simulink library "WECSim_Lib"  (R2014b)
settings: Solver=ode45  StartTime=0.0  StopTime=10.0  RelTol=1e-3
undefined symbols (not defined in the file): body, constraint, pto, simu, waves, X, Y, Z
libraries: nesl_utility x178, sm_lib x59, vrlib x12
(part 2 of 6)

== system WECSim_Lib/Constraints/Heave ==
  note: Constraints the motion to the desired DOF.
      | Moves the connection points (B and F) from the free surface to the PTO location.
      | Outputs forces and motions.
  note: constraint.loc
      | constraint.c
      | constraint.k
      | constraint.name used in mask
  Add : Sum
  "Assignment (3rd index) " : Assignment  Indices=3
  Assignment (3rd index)1 : Assignment  Indices=3
  Assignment (3rd index)2 : Assignment  Indices=3
  Constant{,1..3} (4 alike) : Constant  Value=[0 0 0 0 0 0]
  Initial Displacement and Angle : Constant  Value=constraint.mooring.initLinDispAngle
  Mooring : Subsystem  Variant=on
  Mux : Mux  Inputs=2
  Mux1 : Mux  Inputs=6
  Mux2 : Mux  Inputs=2
  PS-Simulink Converter{,1..6} (7 alike) : nesl_utility/PS-Simulink Converter  PhysicalDomain=network_engine_domain  SubClassName=ps_output  LeftPortType=input  RightPortType=output  PseudoPeriodic=off  Frequencies=[]  Unit=1  AffineConversion=off
  Prismatic Joint (Translational Constraint) : sm_lib/Joints/Prismatic Joint  SenseConstraintForce=on  SenseConstraintForceX=off  SenseConstraintForceY=off  SenseConstraintForceZ=off  SenseConstraintTorque=on  SenseConstraintTorqueX=off  SenseConstraintTorqueY=off  SenseConstraintTorqueZ=off  SenseTotalForce=on  SenseTotalForceX=off  SenseTotalForceY=off  SenseTotalForceZ=off  SenseTotalTorque=on  SenseTotalTorqueX=off  SenseTotalTorqueY=off  SenseTotalTorqueZ=off  CompositeWrenchDir=BaseOnFollower  CompositeWrenchFrame=BaseFrame  EquilibriumPosition=0  EquilibriumPositionUnits=m  SpringStiffness=0  SpringStiffnessUnits=N/m  DampingCoefficient=0  DampingCoefficientUnits=N/(m/s)  TorqueActuationMode=InputTorque  MotionActuationMode=ComputedMotion  SensePosition=on  SenseVelocity=on  SenseAcceleration=on  SenseTorqueForce=off  PositionTargetValue=0  PositionTargetValueUnits=m  PositionTargetSpecify=off  PositionTargetPriority=High  VelocityTargetValue=0  VelocityTargetValueUnits=m/s  VelocityTargetSpecify=off  VelocityTargetPriority=High  BlockFunction=simmechanics.library.joints.prismatic_joint
  Rigid Transform : sm_lib/Frames and Transforms/Rigid Transform  TranslationMethod=Cartesian  TranslationLengthUnit=m  TranslationStandardAxis=+Z  TranslationStandardOffset=0  TranslationCartesianOffset=constraint.loc  TranslationROffset=0  TranslationROffsetUnits=m  TranslationZOffset=0  TranslationZOffsetUnits=m  TranslationThetaOffset=0  TranslationThetaOffsetUnits=deg  RotationMethod=None  RotationAngleUnits=deg  RotationStandardAxis=+X  RotationAngle=90  RotationArbitraryAxis=[0 0 1]  FollAlignAxisA=+X  BaseAlignAxisA=+Y  FollAlignAxisB=+Y  BaseAlignAxisB=+Z  RotationMatrix=[1 0 0; 0 1 0; 0 0 1]  BlockFunction=simmechanics.library.frames_transforms.rigid_transform
  Rigid Transform1 : sm_lib/Frames and Transforms/Rigid Transform  TranslationMethod=Cartesian  TranslationLengthUnit=m  TranslationStandardAxis=+Z  TranslationStandardOffset=0  TranslationCartesianOffset=constraint.loc  TranslationROffset=0  TranslationROffsetUnits=m  TranslationZOffset=0  TranslationZOffsetUnits=m  TranslationThetaOffset=0  TranslationThetaOffsetUnits=deg  RotationMethod=None  RotationAngleUnits=deg  RotationStandardAxis=+X  RotationAngle=90  RotationArbitraryAxis=[0 0 1]  FollAlignAxisA=+X  BaseAlignAxisA=+Y  FollAlignAxisB=+Y  BaseAlignAxisB=+Z  RotationMatrix=[1 0 0; 0 1 0; 0 0 1]  BlockFunction=simmechanics.library.frames_transforms.rigid_transform
  Selector2 : Selector  InputPortWidth=6  Indices=3
  Simulink-PS Converter2 : nesl_utility/Simulink-PS Converter  PhysicalDomain=network_engine_domain  SubClassName=ps_input  LeftPortType=input  RightPortType=output  PseudoPeriodic=off  Frequencies=[]  NoiseDistribution=none  NoiseParameters=[]  Unit=1  AffineConversion=off  InputFiltering=off  SimscapeFilterOrder=1  InputFilterTimeConstant=0.001  UdotUserProvided=1
  output : ToWorkspace  VariableName=constraint1_out  SaveFormat=Structure With Time  SampleTime=-1
      settings: Decimation=round(simu.dtOut/simu.dt,0)
  F : PMIOPort  Port=1  Side=Right
  B : PMIOPort  Port=2  Side=Left
  wires:
  Mux1/1 -> output/1
  Assignment (3rd index)2/1 -> Mux1/3  "acceleration"
  Constant/1 -> "Assignment (3rd index) "/1
  PS-Simulink Converter2/1 -> "Assignment (3rd index) "/2
  Constant1/1 -> Assignment (3rd index)1/1
  PS-Simulink Converter3/1 -> Assignment (3rd index)1/2
  Constant2/1 -> Assignment (3rd index)2/1
  PS-Simulink Converter4/1 -> Assignment (3rd index)2/2
  Mux/1 -> Mux1/5  "Constraint Forces"
  PS-Simulink Converter1/1 -> Mux/2
  PS-Simulink Converter/1 -> Mux/1
  Mux2/1 -> Mux1/4  "Total Forces"
  PS-Simulink Converter6/1 -> Mux2/2
  PS-Simulink Converter5/1 -> Mux2/1
  Constant3/1 -> Mux1/6  "Mooring Forces"
  Assignment (3rd index)1/1 -> Mooring/3(Velocity), Mux1/2  "velocity"
  "Assignment (3rd index) "/1 -> Add/1, Mux1/1  "position"
  Mooring/1(F_Mooring) -> Selector2/1
  Selector2/1 -> Simulink-PS Converter2/1
  [Clock] -> Mooring/2(Clock)
  Initial Displacement and Angle/1 -> Add/2
  Add/1 -> Mooring/1(Displacement)
  connections:
  PS-Simulink Converter1/LConn1 -- Prismatic Joint (Translational Constraint)/RConn6
  Prismatic Joint (Translational Constraint)/RConn5 -- PS-Simulink Converter/LConn1
  PS-Simulink Converter4/LConn1 -- Prismatic Joint (Translational Constraint)/RConn4
  PS-Simulink Converter3/LConn1 -- Prismatic Joint (Translational Constraint)/RConn3
  PS-Simulink Converter2/LConn1 -- Prismatic Joint (Translational Constraint)/RConn2
  Rigid Transform/RConn1 -- Prismatic Joint (Translational Constraint)/LConn1
  B/RConn1 -- Rigid Transform/LConn1
  Rigid Transform1/LConn1 -- F/RConn1
  Rigid Transform1/RConn1 -- Prismatic Joint (Translational Constraint)/RConn1
  Prismatic Joint (Translational Constraint)/RConn7 -- PS-Simulink Converter5/LConn1
  Prismatic Joint (Translational Constraint)/RConn8 -- PS-Simulink Converter6/LConn1
  Simulink-PS Converter2/RConn1 -- Prismatic Joint (Translational Constraint)/LConn2

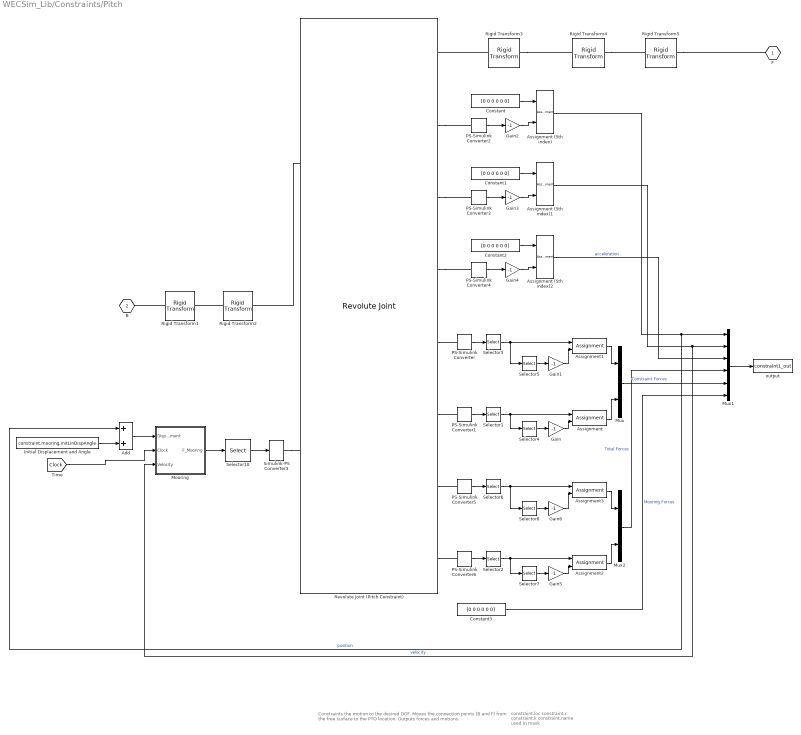
== system WECSim_Lib/Constraints/Pitch ==
  note: constraint.loc
      | constraint.c
      | constraint.k
      | constraint.name used in mask
  note: Constraints the motion to the desired DOF.
      | Moves the connection points (B and F) from the free surface to the PTO location.
      | Outputs forces and motions.
  Add : Sum
  Assignment{,1..3} (4 alike) : Assignment  DiagnosticForDimensions=Warning  Indices=2
  "Assignment (5th index) " : Assignment  Indices=5
  Assignment (5th index)1 : Assignment  Indices=5
  Assignment (5th index)2 : Assignment  Indices=5
  Constant{,1..3} (4 alike) : Constant  Value=[0 0 0 0 0 0]
  Gain{,1..6} (7 alike) : Gain  Gain=-1
  Initial Displacement and Angle : Constant  Value=constraint.mooring.initLinDispAngle
  Mooring : Subsystem  Variant=on
  Mux : Mux  Inputs=2
  Mux1 : Mux  Inputs=6
  Mux2 : Mux  Inputs=2
  PS-Simulink Converter{,1..6} (7 alike) : nesl_utility/PS-Simulink Converter  PhysicalDomain=network_engine_domain  SubClassName=ps_output  LeftPortType=input  RightPortType=output  PseudoPeriodic=off  Frequencies=[]  Unit=1  AffineConversion=off
  Revolute Joint (Pitch Constraint) : sm_lib/Joints/Revolute Joint  SenseConstraintForce=on  SenseConstraintForceX=off  SenseConstraintForceY=off  SenseConstraintForceZ=off  SenseConstraintTorque=on  SenseConstraintTorqueX=off  SenseConstraintTorqueY=off  SenseConstraintTorqueZ=off  SenseTotalForce=on  SenseTotalForceX=off  SenseTotalForceY=off  SenseTotalForceZ=off  SenseTotalTorque=on  SenseTotalTorqueX=off  SenseTotalTorqueY=off  SenseTotalTorqueZ=off  CompositeWrenchDir=BaseOnFollower  CompositeWrenchFrame=BaseFrame  EquilibriumPosition=0  EquilibriumPositionUnits=deg  SpringStiffness=0  SpringStiffnessUnits=N*m/deg  DampingCoefficient=0  DampingCoefficientUnits=N*m/(rad/s)  TorqueActuationMode=InputTorque  MotionActuationMode=ComputedMotion  SensePosition=on  SenseVelocity=on  SenseAcceleration=on  SenseTorqueForce=off  PositionTargetValue=0  PositionTargetValueUnits=deg  PositionTargetSpecify=off  PositionTargetPriority=High  VelocityTargetValue=0  VelocityTargetValueUnits=deg/s  VelocityTargetSpecify=off  VelocityTargetPriority=High  BlockFunction=simmechanics.library.joints.revolute_joint
  Rigid Transform1 : sm_lib/Frames and Transforms/Rigid Transform  TranslationMethod=Cartesian  TranslationLengthUnit=m  TranslationStandardAxis=+Z  TranslationStandardOffset=0  TranslationCartesianOffset=constraint.loc  TranslationROffset=0  TranslationROffsetUnits=m  TranslationZOffset=0  TranslationZOffsetUnits=m  TranslationThetaOffset=0  TranslationThetaOffsetUnits=deg  RotationMethod=None  RotationAngleUnits=deg  RotationStandardAxis=+X  RotationAngle=90  RotationArbitraryAxis=[0 0 1]  FollAlignAxisA=+X  BaseAlignAxisA=+Y  FollAlignAxisB=+Y  BaseAlignAxisB=+Z  RotationMatrix=[1 0 0; 0 1 0; 0 0 1]  BlockFunction=simmechanics.library.frames_transforms.rigid_transform
  Rigid Transform2 : sm_lib/Frames and Transforms/Rigid Transform  TranslationMethod=None  TranslationLengthUnit=m  TranslationStandardAxis=+Z  TranslationStandardOffset=0  TranslationCartesianOffset=[0 0 0]  TranslationROffset=0  TranslationROffsetUnits=m  TranslationZOffset=0  TranslationZOffsetUnits=m  TranslationThetaOffset=0  TranslationThetaOffsetUnits=deg  RotationMethod=StandardAxis  RotationAngleUnits=deg  RotationStandardAxis=+X  RotationAngle=90  RotationArbitraryAxis=[0 0 1]  FollAlignAxisA=+X  BaseAlignAxisA=+Y  FollAlignAxisB=+Y  BaseAlignAxisB=+Z  RotationMatrix=[1 0 0; 0 1 0; 0 0 1]  BlockFunction=simmechanics.library.frames_transforms.rigid_transform
  Rigid Transform3 : sm_lib/Frames and Transforms/Rigid Transform  TranslationMethod=None  TranslationLengthUnit=m  TranslationStandardAxis=+Z  TranslationStandardOffset=0  TranslationCartesianOffset=constraint.loc  TranslationROffset=0  TranslationROffsetUnits=m  TranslationZOffset=0  TranslationZOffsetUnits=m  TranslationThetaOffset=0  TranslationThetaOffsetUnits=deg  RotationMethod=StandardAxis  RotationAngleUnits=rad  RotationStandardAxis=-Z  RotationAngle=constraint.initDisp  RotationArbitraryAxis=[0 0 1]  FollAlignAxisA=+X  BaseAlignAxisA=+Y  FollAlignAxisB=+Y  BaseAlignAxisB=+Z  RotationMatrix=[1 0 0; 0 1 0; 0 0 1]  BlockFunction=simmechanics.library.frames_transforms.rigid_transform
  Rigid Transform4 : sm_lib/Frames and Transforms/Rigid Transform  TranslationMethod=None  TranslationLengthUnit=m  TranslationStandardAxis=+Z  TranslationStandardOffset=0  TranslationCartesianOffset=constraint.loc  TranslationROffset=0  TranslationROffsetUnits=m  TranslationZOffset=0  TranslationZOffsetUnits=m  TranslationThetaOffset=0  TranslationThetaOffsetUnits=deg  RotationMethod=StandardAxis  RotationAngleUnits=deg  RotationStandardAxis=+X  RotationAngle=-90  RotationArbitraryAxis=[0 0 1]  FollAlignAxisA=+X  BaseAlignAxisA=+Y  FollAlignAxisB=+Y  BaseAlignAxisB=+Z  RotationMatrix=[1 0 0; 0 1 0; 0 0 1]  BlockFunction=simmechanics.library.frames_transforms.rigid_transform
  Rigid Transform5 : sm_lib/Frames and Transforms/Rigid Transform  TranslationMethod=Cartesian  TranslationLengthUnit=m  TranslationStandardAxis=+Z  TranslationStandardOffset=0  TranslationCartesianOffset=[-constraint.loc(1)*cos(-constraint.initDisp)-constraint.loc(3)*sin(-constraint.initDisp), 0, constraint.loc(1)*sin(-constraint.initDisp)-constraint.loc(3)*cos(-constraint.initDisp)]  TranslationROffset=0  TranslationROffsetUnits=m  TranslationZOffset=0  TranslationZOffsetUnits=m  TranslationThetaOffset=0  TranslationThetaOffsetUnits=deg  RotationMethod=None  RotationAngleUnits=deg  RotationStandardAxis=+X  RotationAngle=-90  RotationArbitraryAxis=[0 0 1]  FollAlignAxisA=+X  BaseAlignAxisA=+Y  FollAlignAxisB=+Y  BaseAlignAxisB=+Z  RotationMatrix=[1 0 0; 0 1 0; 0 0 1]  BlockFunction=simmechanics.library.frames_transforms.rigid_transform
  Selector{1..3,6} (4 alike) : Selector  InputPortWidth=3  Indices=[1 3 2]
  Selector10 : Selector  InputPortWidth=6  Indices=5
  Selector{4..5,7..8} (4 alike) : Selector  InputPortWidth=3  Indices=[2]
  Simulink-PS Converter3 : nesl_utility/Simulink-PS Converter  PhysicalDomain=network_engine_domain  SubClassName=ps_input  LeftPortType=input  RightPortType=output  PseudoPeriodic=off  Frequencies=[]  NoiseDistribution=none  NoiseParameters=[]  Unit=1  AffineConversion=off  InputFiltering=off  SimscapeFilterOrder=1  InputFilterTimeConstant=0.001  UdotUserProvided=1
  output : ToWorkspace  VariableName=constraint1_out  SaveFormat=Structure With Time  SampleTime=-1
      settings: Decimation=round(simu.dtOut/simu.dt,0)
  F : PMIOPort  Port=1  Side=Right
  B : PMIOPort  Port=2  Side=Left
  wires:
  Constant3/1 -> Mux1/6  "Mooring Forces"
  PS-Simulink Converter5/1 -> Selector6/1
  PS-Simulink Converter6/1 -> Selector2/1
  Selector2/1 -> Assignment2/1, Selector7/1
  Selector7/1 -> Gain5/1
  Gain5/1 -> Assignment2/2
  Selector6/1 -> Assignment3/1, Selector8/1
  Selector8/1 -> Gain6/1
  Gain6/1 -> Assignment3/2
  Assignment3/1 -> Mux2/1
  Assignment2/1 -> Mux2/2
  Mux2/1 -> Mux1/4  "Total Forces"
  PS-Simulink Converter/1 -> Selector3/1
  PS-Simulink Converter1/1 -> Selector1/1
  Selector1/1 -> Selector4/1, Assignment/1
  Selector4/1 -> Gain/1
  Gain/1 -> Assignment/2
  Selector3/1 -> Selector5/1, Assignment1/1
  Selector5/1 -> Gain1/1
  Gain1/1 -> Assignment1/2
  Assignment1/1 -> Mux/1
  Assignment (5th index)2/1 -> Mux1/3  "acceleration"
  Gain4/1 -> Assignment (5th index)2/2
  Constant2/1 -> Assignment (5th index)2/1
  PS-Simulink Converter4/1 -> Gain4/1
  PS-Simulink Converter3/1 -> Gain3/1
  Gain3/1 -> Assignment (5th index)1/2
  Constant1/1 -> Assignment (5th index)1/1
  Gain2/1 -> "Assignment (5th index) "/2
  PS-Simulink Converter2/1 -> Gain2/1
  Constant/1 -> "Assignment (5th index) "/1
  Assignment/1 -> Mux/2
  Mux1/1 -> output/1
  Mux/1 -> Mux1/5  "Constraint Forces"
  Assignment (5th index)1/1 -> Mooring/3(Velocity), Mux1/2  "velocity"
  "Assignment (5th index) "/1 -> Add/1, Mux1/1  "position"
  Mooring/1(F_Mooring) -> Selector10/1
  Selector10/1 -> Simulink-PS Converter3/1
  [Clock] -> Mooring/2(Clock)
  Initial Displacement and Angle/1 -> Add/2
  Add/1 -> Mooring/1(Displacement)
  connections:
  Rigid Transform5/RConn1 -- F/RConn1
  Rigid Transform4/RConn1 -- Rigid Transform5/LConn1
  Rigid Transform3/RConn1 -- Rigid Transform4/LConn1
  PS-Simulink Converter6/LConn1 -- Revolute Joint (Pitch Constraint)/RConn8
  PS-Simulink Converter5/LConn1 -- Revolute Joint (Pitch Constraint)/RConn7
  Rigid Transform2/LConn1 -- Rigid Transform1/RConn1
  Revolute Joint (Pitch Constraint)/LConn1 -- Rigid Transform2/RConn1
  PS-Simulink Converter/LConn1 -- Revolute Joint (Pitch Constraint)/RConn5
  PS-Simulink Converter1/LConn1 -- Revolute Joint (Pitch Constraint)/RConn6
  Revolute Joint (Pitch Constraint)/RConn2 -- PS-Simulink Converter2/LConn1
  Revolute Joint (Pitch Constraint)/RConn3 -- PS-Simulink Converter3/LConn1
  Revolute Joint (Pitch Constraint)/RConn4 -- PS-Simulink Converter4/LConn1
  Rigid Transform3/LConn1 -- Revolute Joint (Pitch Constraint)/RConn1
  Rigid Transform1/LConn1 -- B/RConn1
  Simulink-PS Converter3/RConn1 -- Revolute Joint (Pitch Constraint)/LConn2

== system WECSim_Lib/Constraints/Surge ==
  note: Constraints the motion to the desired DOF.
      | Moves the connection points (B and F) from the free surface to the PTO location.
      | Outputs forces and motions.
  note: constraint.loc
      | constraint.c
      | constraint.k
      | constraint.name used in mask
  Add : Sum
  Assignment{,1..3} (4 alike) : Assignment  DiagnosticForDimensions=Warning  Indices=3
  "Assignment (1st index) " : Assignment
  Assignment (1st index)1 : Assignment
  Assignment (1st index)2 : Assignment
  Constant{,1..3} (4 alike) : Constant  Value=[0 0 0 0 0 0]
  Gain{,1..3} (4 alike) : Gain  Gain=-1
  Initial Displacement and Angle : Constant  Value=constraint.mooring.initLinDispAngle
  Mooring : Subsystem  Variant=on
  Mux : Mux  Inputs=2
  Mux1 : Mux  Inputs=6
  Mux2 : Mux  Inputs=2
  PS-Simulink Converter{1..7} (7 alike) : nesl_utility/PS-Simulink Converter  PhysicalDomain=network_engine_domain  SubClassName=ps_output  LeftPortType=input  RightPortType=output  PseudoPeriodic=off  Frequencies=[]  Unit=1  AffineConversion=off
  Prismatic Joint (Translational Constraint) : sm_lib/Joints/Prismatic Joint  SenseConstraintForce=on  SenseConstraintForceX=off  SenseConstraintForceY=off  SenseConstraintForceZ=off  SenseConstraintTorque=on  SenseConstraintTorqueX=off  SenseConstraintTorqueY=off  SenseConstraintTorqueZ=off  SenseTotalForce=on  SenseTotalForceX=off  SenseTotalForceY=off  SenseTotalForceZ=off  SenseTotalTorque=on  SenseTotalTorqueX=off  SenseTotalTorqueY=off  SenseTotalTorqueZ=off  CompositeWrenchDir=BaseOnFollower  CompositeWrenchFrame=BaseFrame  EquilibriumPosition=0  EquilibriumPositionUnits=m  SpringStiffness=0  SpringStiffnessUnits=N/m  DampingCoefficient=0  DampingCoefficientUnits=N/(m/s)  TorqueActuationMode=InputTorque  MotionActuationMode=ComputedMotion  SensePosition=on  SenseVelocity=on  SenseAcceleration=on  SenseTorqueForce=off  PositionTargetValue=0  PositionTargetValueUnits=m  PositionTargetSpecify=off  PositionTargetPriority=High  VelocityTargetValue=0  VelocityTargetValueUnits=m/s  VelocityTargetSpecify=off  VelocityTargetPriority=High  BlockFunction=simmechanics.library.joints.prismatic_joint
  Rigid Transform : sm_lib/Frames and Transforms/Rigid Transform  TranslationMethod=Cartesian  TranslationLengthUnit=m  TranslationStandardAxis=+Z  TranslationStandardOffset=0  TranslationCartesianOffset=constraint.loc  TranslationROffset=0  TranslationROffsetUnits=m  TranslationZOffset=0  TranslationZOffsetUnits=m  TranslationThetaOffset=0  TranslationThetaOffsetUnits=deg  RotationMethod=StandardAxis  RotationAngleUnits=deg  RotationStandardAxis=+Y  RotationAngle=90  RotationArbitraryAxis=[0 0 1]  FollAlignAxisA=+X  BaseAlignAxisA=+Y  FollAlignAxisB=+Y  BaseAlignAxisB=+Z  RotationMatrix=[1 0 0; 0 1 0; 0 0 1]  BlockFunction=simmechanics.library.frames_transforms.rigid_transform
  Rigid Transform1 : sm_lib/Frames and Transforms/Rigid Transform  TranslationMethod=Cartesian  TranslationLengthUnit=m  TranslationStandardAxis=+Z  TranslationStandardOffset=0  TranslationCartesianOffset=constraint.loc  TranslationROffset=0  TranslationROffsetUnits=m  TranslationZOffset=0  TranslationZOffsetUnits=m  TranslationThetaOffset=0  TranslationThetaOffsetUnits=deg  RotationMethod=StandardAxis  RotationAngleUnits=deg  RotationStandardAxis=+Y  RotationAngle=90  RotationArbitraryAxis=[0 0 1]  FollAlignAxisA=+X  BaseAlignAxisA=+Y  FollAlignAxisB=+Y  BaseAlignAxisB=+Z  RotationMatrix=[1 0 0; 0 1 0; 0 0 1]  BlockFunction=simmechanics.library.frames_transforms.rigid_transform
  Selector : Selector  InputPortWidth=6
  Selector{1..2,5..6} (4 alike) : Selector  InputPortWidth=3  Indices=[3 2 1]
  Selector{3..4,7..8} (4 alike) : Selector  InputPortWidth=3  Indices=[3]
  Simulink-PS Converter1 : nesl_utility/Simulink-PS Converter  PhysicalDomain=network_engine_domain  SubClassName=ps_input  LeftPortType=input  RightPortType=output  PseudoPeriodic=off  Frequencies=[]  NoiseDistribution=none  NoiseParameters=[]  Unit=1  AffineConversion=off  InputFiltering=off  SimscapeFilterOrder=1  InputFilterTimeConstant=0.001  UdotUserProvided=1
  output : ToWorkspace  VariableName=constraint1_out  SaveFormat=Structure With Time  SampleTime=-1
      settings: Decimation=round(simu.dtOut/simu.dt,0)
  F : PMIOPort  Port=1  Side=Right
  B : PMIOPort  Port=2  Side=Left
  wires:
  Mux1/1 -> output/1
  Assignment (1st index)2/1 -> Mux1/3  "acceleration"
  Constant/1 -> "Assignment (1st index) "/1
  PS-Simulink Converter2/1 -> "Assignment (1st index) "/2
  Constant1/1 -> Assignment (1st index)1/1
  PS-Simulink Converter3/1 -> Assignment (1st index)1/2
  Constant2/1 -> Assignment (1st index)2/1
  PS-Simulink Converter4/1 -> Assignment (1st index)2/2
  PS-Simulink Converter5/1 -> Selector2/1
  PS-Simulink Converter1/1 -> Selector1/1
  Assignment1/1 -> Mux/1
  Assignment/1 -> Mux/2
  Gain1/1 -> Assignment1/2
  Selector3/1 -> Gain1/1
  Selector2/1 -> Assignment1/1, Selector3/1
  Gain/1 -> Assignment/2
  Selector4/1 -> Gain/1
  Selector1/1 -> Assignment/1, Selector4/1
  Mux/1 -> Mux1/5  "Constraint Forces"
  Constant3/1 -> Mux1/6  "Mooring Forces"
  PS-Simulink Converter7/1 -> Selector6/1
  PS-Simulink Converter6/1 -> Selector5/1
  Assignment3/1 -> Mux2/1
  Assignment2/1 -> Mux2/2
  Gain3/1 -> Assignment3/2
  Selector7/1 -> Gain3/1
  Selector6/1 -> Assignment3/1, Selector7/1
  Gain2/1 -> Assignment2/2
  Selector8/1 -> Gain2/1
  Selector5/1 -> Assignment2/1, Selector8/1
  Mux2/1 -> Mux1/4  "Total Forces"
  Assignment (1st index)1/1 -> Mooring/3(Velocity), Mux1/2  "velocity"
  "Assignment (1st index) "/1 -> Add/1, Mux1/1  "position"
  Mooring/1(F_Mooring) -> Selector/1
  [Clock] -> Mooring/2(Clock)
  Initial Displacement and Angle/1 -> Add/2
  Add/1 -> Mooring/1(Displacement)
  Selector/1 -> Simulink-PS Converter1/1
  connections:
  F/RConn1 -- Rigid Transform1/LConn1
  PS-Simulink Converter1/LConn1 -- Prismatic Joint (Translational Constraint)/RConn6
  PS-Simulink Converter5/LConn1 -- Prismatic Joint (Translational Constraint)/RConn5
  PS-Simulink Converter2/LConn1 -- Prismatic Joint (Translational Constraint)/RConn2
  PS-Simulink Converter3/LConn1 -- Prismatic Joint (Translational Constraint)/RConn3
  PS-Simulink Converter4/LConn1 -- Prismatic Joint (Translational Constraint)/RConn4
  Rigid Transform/LConn1 -- B/RConn1
  Rigid Transform/RConn1 -- Prismatic Joint (Translational Constraint)/LConn1
  Rigid Transform1/RConn1 -- Prismatic Joint (Translational Constraint)/RConn1
  Prismatic Joint (Translational Constraint)/RConn7 -- PS-Simulink Converter7/LConn1
  Prismatic Joint (Translational Constraint)/RConn8 -- PS-Simulink Converter6/LConn1
  Simulink-PS Converter1/RConn1 -- Prismatic Joint (Translational Constraint)/LConn2

== system WECSim_Lib/Frames/Global Reference Frame ==
  note: simu.domainSize
      | waves.waterDepth
  note: Serves as the global reference frame for any WEC-Sim simulation.
      | Has a connection point at (0,0,0), defined at the free surface.
      | Sets up the free surface and ground visualization.
      | Sends the simulation time to a GoTo that can be accesed by other blocks.
  Clock : Clock
  Mean Free Surface : sm_lib/Body Elements/Solid  InertiaType=Custom  Mass=10^20  MassUnits=kg  CenterOfMass=[0 0 0]  CenterOfMassUnits=m  MomentsOfInertia=[10^20 10^20 10^20]  MomentsOfInertiaUnits=kg*m^2  ProductsOfInertia=[0 0 0]  ProductsOfInertiaUnits=kg*m^2  DensityBased=on  Density=1000  DensityUnits=kg/(m^3)  GraphicType=FromGeometry  MarkerShape=Sphere  MarkerSize=10  MarkerSizeUnits=m  GraphicVisPropType=SimpleVisualProperties  GraphicDiffuseColor=[0.0 0.6 0.8]  GraphicSpecularColor=[0.5 0.5 0.5 1.0]  GraphicAmbientColor=[0.15 0.15 0.15 1.0]  GraphicEmissiveColor=[0.0 0.0 0.0 1.0]  GraphicShininess=75  GraphicOpacity=0.3  GeometryShape=GeneralExtrusion  RectangleSize=[1 1]  RectangleSizeUnits=m  BrickDimensions=[1 1 1]  BrickDimensionUnits=m  CylinderRadius=1  CylinderRadiusUnits=m  CylinderLength=1  CylinderLengthUnits=m  SphereRadius=1  SphereRadiusUnits=m  EllipsoidRadii=[1 1 1]  EllipsoidRadiiUnits=m  ExtrusionCrossSection=[simu.domainSize simu.domainSize; -simu.domainSize simu.domainSize; -simu.domainSize -simu.domainSize; simu.domainSize -simu.domainSize]  ExtrusionCrossSectionUnits=m  ExtrusionLength=simu.domainSize/200  ExtrusionLengthUnits=m  PolygonNumSides=3  PolygonOuterRadius=1  PolygonOuterRadiusUnits=m  ExtGeomFileType=STL  ExtGeomFileUnits=m  RevolutionCrossSection=[1 1; 1 -1; 2 -1; 2 1]  RevolutionCrossSectionUnits=m  RevolutionExtent=Full  RevolutionAngle=180  RevolutionAngleUnits=deg  BlockFunction=simmechanics.library.body_elements.solid
  Mechanism Configuration : sm_lib/Utilities/Mechanism Configuration  UniformGravity=Constant  GravityVector=[0 0 0]  GravityUnits=m/s^2  LinearizationDelta=0.001  BlockFunction=simmechanics.library.utilities.mechanism_configuration
  Rigid Transform : sm_lib/Frames and Transforms/Rigid Transform  TranslationMethod=Cartesian  TranslationLengthUnit=m  TranslationStandardAxis=+Z  TranslationStandardOffset=0  TranslationCartesianOffset=[0 0 -waves.waterDepth]  TranslationROffset=0  TranslationROffsetUnits=m  TranslationZOffset=0  TranslationZOffsetUnits=m  TranslationThetaOffset=0  TranslationThetaOffsetUnits=deg  RotationMethod=None  RotationAngleUnits=deg  RotationStandardAxis=+Z  RotationAngle=0  RotationArbitraryAxis=[0 0 1]  FollAlignAxisA=+X  BaseAlignAxisA=+Y  FollAlignAxisB=+Y  BaseAlignAxisB=+Z  RotationMatrix=[1 0 0; 0 1 0; 0 0 1]  BlockFunction=simmechanics.library.frames_transforms.rigid_transform
  Seabed : sm_lib/Body Elements/Solid  InertiaType=Custom  Mass=10^20  MassUnits=kg  CenterOfMass=[0 0 0]  CenterOfMassUnits=m  MomentsOfInertia=[10^20 10^20 10^20]  MomentsOfInertiaUnits=kg*m^2  ProductsOfInertia=[0 0 0]  ProductsOfInertiaUnits=kg*m^2  DensityBased=on  Density=1000  DensityUnits=kg/(m^3)  GraphicType=FromGeometry  MarkerShape=Sphere  MarkerSize=10  MarkerSizeUnits=m  GraphicVisPropType=SimpleVisualProperties  GraphicDiffuseColor=[0.4 0.4 0.0]  GraphicSpecularColor=[0.5 0.5 0.5 1.0]  GraphicAmbientColor=[0.15 0.15 0.15 1.0]  GraphicEmissiveColor=[0.0 0.0 0.0 1.0]  GraphicShininess=75  GraphicOpacity=1  GeometryShape=GeneralExtrusion  RectangleSize=[1 1]  RectangleSizeUnits=m  BrickDimensions=[1 1 1]  BrickDimensionUnits=m  CylinderRadius=1  CylinderRadiusUnits=m  CylinderLength=1  CylinderLengthUnits=m  SphereRadius=1  SphereRadiusUnits=m  EllipsoidRadii=[1 1 1]  EllipsoidRadiiUnits=m  ExtrusionCrossSection=[simu.domainSize simu.domainSize; -simu.domainSize simu.domainSize; -simu.domainSize -simu.domainSize; simu.domainSize -simu.domainSize]  ExtrusionCrossSectionUnits=m  ExtrusionLength=simu.domainSize/100  ExtrusionLengthUnits=m  PolygonNumSides=3  PolygonOuterRadius=1  PolygonOuterRadiusUnits=m  ExtGeomFileType=STL  ExtGeomFileUnits=m  RevolutionCrossSection=[1 1; 1 -1; 2 -1; 2 1]  RevolutionCrossSectionUnits=m  RevolutionExtent=Full  RevolutionAngle=180  RevolutionAngleUnits=deg  BlockFunction=simmechanics.library.body_elements.solid
  Solver Configuration : nesl_utility/Solver Configuration  PhysicalDomain=network_engine_domain  SubClassName=solver  LeftPortType=input  RightPortType=generic  Accelerate=off  Tones=[]  Harmonics=[]  SimulateNoise=off  Profile=off  UseLocalSampling=off  EnableSwitchedLinearOptims=on  FrequencyDomain=off  UseCCode=off  RelTol=0.001  AbsTol=1e-06  MinStep=1e-09  ToWorkspace=off  DoDC=on  ResidualTolerance=1e-9  UseLocalSolver=off  LocalSolverChoice=NE_BACKWARD_EULER_ADVANCER  LocalSolverSampleTime=.001  DoFixedCost=off  MaxNonlinIter=3  MaxModeIter=2  LinearAlgebra=Sparse  DelaysMemoryBudget=1024  AutomaticFiltering=on  FilteringTimeConstant=0.001
  World Frame : sm_lib/Frames and Transforms/World Frame  BlockFunction=simmechanics.library.frames_transforms.world_frame
  Conn : PMIOPort  Port=1  Side=Right
  tag scope: Clock=global
  wires:
  Clock/1 -> [Clock]
  connections:
  Mechanism Configuration/RConn1 -- World Frame/RConn1 -- Solver Configuration/RConn1 -- Conn/RConn1 -- Mean Free Surface/RConn1 -- Rigid Transform/LConn1
  Seabed/RConn1 -- Rigid Transform/RConn1

== system WECSim_Lib/PTOs/Rotational PTO (Local RY) ==
  note: pto.loc
      | pto.c
      | pto.k
  note: Constraints the motion to the desired DOF.
      | Applies PTO loads to the body based on PTO restoring and damping values.
      | Moves the connection points (B and F) from the free surface to the PTO location.
      | Calculates the PTO internal mecahnics force and power.
      | Outputs motions, forces, and power.
  Assignment{,1..3} (4 alike) : Assignment  DiagnosticForDimensions=Warning  Indices=2
  "Assignment (5th index) " : Assignment  Indices=5
  Assignment (5th index)1 : Assignment  Indices=5
  Assignment (5th index)2 : Assignment  Indices=5
  Assignment (5th index)3 : Assignment  Indices=5
  Bus Creator1 : BusCreator  Inputs=8
  Constant{,1..3} (4 alike) : Constant  Value=[0 0 0 0 0 0]
  Gain{,1..7} (8 alike) : Gain  Gain=-1
  InternalMechanics : Subsystem
  Mux1 : Mux  Inputs=2
  Mux4 : Mux  Inputs=2
  PS-Simulink Converter{,1..7} (8 alike) : nesl_utility/PS-Simulink Converter  PhysicalDomain=network_engine_domain  SubClassName=ps_output  LeftPortType=input  RightPortType=output  PseudoPeriodic=off  Frequencies=[]  Unit=1  AffineConversion=off
  Pitch PCC (Revolute Joint) : sm_lib/Joints/Revolute Joint  SenseConstraintForce=on  SenseConstraintForceX=off  SenseConstraintForceY=off  SenseConstraintForceZ=off  SenseConstraintTorque=on  SenseConstraintTorqueX=off  SenseConstraintTorqueY=off  SenseConstraintTorqueZ=off  SenseTotalForce=on  SenseTotalForceX=off  SenseTotalForceY=off  SenseTotalForceZ=off  SenseTotalTorque=on  SenseTotalTorqueX=off  SenseTotalTorqueY=off  SenseTotalTorqueZ=off  CompositeWrenchDir=BaseOnFollower  CompositeWrenchFrame=BaseFrame  EquilibriumPosition=0  EquilibriumPositionUnits=deg  SpringStiffness=pto.k  SpringStiffnessUnits=N*m/rad  DampingCoefficient=pto.c  DampingCoefficientUnits=N*m/(rad/s)  TorqueActuationMode=NoTorque  MotionActuationMode=ComputedMotion  SensePosition=on  SenseVelocity=on  SenseAcceleration=on  SenseTorqueForce=on  PositionTargetValue=0  PositionTargetValueUnits=deg  PositionTargetSpecify=off  PositionTargetPriority=High  VelocityTargetValue=0  VelocityTargetValueUnits=deg/s  VelocityTargetSpecify=off  VelocityTargetPriority=High  BlockFunction=simmechanics.library.joints.revolute_joint
  Rigid Transform : sm_lib/Frames and Transforms/Rigid Transform  TranslationMethod=Cartesian  TranslationLengthUnit=m  TranslationStandardAxis=+Z  TranslationStandardOffset=0  TranslationCartesianOffset=pto.loc  TranslationROffset=0  TranslationROffsetUnits=m  TranslationZOffset=0  TranslationZOffsetUnits=m  TranslationThetaOffset=0  TranslationThetaOffsetUnits=deg  RotationMethod=StandardAxis  RotationAngleUnits=deg  RotationStandardAxis=+X  RotationAngle=90  RotationArbitraryAxis=[0 0 1]  FollAlignAxisA=+X  BaseAlignAxisA=+Y  FollAlignAxisB=+Y  BaseAlignAxisB=+Z  RotationMatrix=[1 0 0; 0 1 0; 0 0 1]  BlockFunction=simmechanics.library.frames_transforms.rigid_transform
  Rigid Transform1 : sm_lib/Frames and Transforms/Rigid Transform  TranslationMethod=Cartesian  TranslationLengthUnit=m  TranslationStandardAxis=+Z  TranslationStandardOffset=0  TranslationCartesianOffset=pto.loc  TranslationROffset=0  TranslationROffsetUnits=m  TranslationZOffset=0  TranslationZOffsetUnits=m  TranslationThetaOffset=0  TranslationThetaOffsetUnits=deg  RotationMethod=StandardAxis  RotationAngleUnits=deg  RotationStandardAxis=+X  RotationAngle=90  RotationArbitraryAxis=[0 0 1]  FollAlignAxisA=+X  BaseAlignAxisA=+Y  FollAlignAxisB=+Y  BaseAlignAxisB=+Z  RotationMatrix=[1 0 0; 0 1 0; 0 0 1]  BlockFunction=simmechanics.library.frames_transforms.rigid_transform
  Selector{,2,4,6} (4 alike) : Selector  InputPortWidth=3  Indices=[1 3 2]
  Selector{1,3,5,7} (4 alike) : Selector  InputPortWidth=3  Indices=[2]
  output : ToWorkspace  VariableName=pto1_out  SaveFormat=Structure With Time  SampleTime=-1
      settings: Decimation=round(simu.dtOut/simu.dt,0)
  F : PMIOPort  Port=1  Side=Right
  B : PMIOPort  Port=2  Side=Left
  wires:
  Selector2/1 -> Assignment/1, Selector3/1
  Selector3/1 -> Gain5/1
  Gain5/1 -> Assignment/2
  Selector/1 -> Assignment1/1, Selector1/1
  Selector1/1 -> Gain4/1
  Gain4/1 -> Assignment1/2
  Assignment/1 -> Mux1/2
  Assignment1/1 -> Mux1/1
  Mux1/1 -> Bus Creator1/6  "forceConstraint"
  PS-Simulink Converter5/1 -> Selector2/1
  PS-Simulink Converter4/1 -> Selector/1
  Bus Creator1/1 -> output/1
  Mux4/1 -> Bus Creator1/4  "forceTotal"
  Selector6/1 -> Selector7/1, Assignment2/1
  Selector7/1 -> Gain7/1
  Gain7/1 -> Assignment2/2
  Selector4/1 -> Selector5/1, Assignment3/1
  Selector5/1 -> Gain6/1
  Gain6/1 -> Assignment3/2
  PS-Simulink Converter6/1 -> Selector4/1
  PS-Simulink Converter7/1 -> Selector6/1
  Assignment2/1 -> Mux4/2
  Assignment3/1 -> Mux4/1
  Constant/1 -> "Assignment (5th index) "/1
  PS-Simulink Converter/1 -> Gain/1
  Gain/1 -> "Assignment (5th index) "/2
  "Assignment (5th index) "/1 -> InternalMechanics/1(Position), Bus Creator1/1  "position"
  Constant1/1 -> Assignment (5th index)1/1
  Gain1/1 -> Assignment (5th index)1/2
  PS-Simulink Converter1/1 -> Gain1/1
  Assignment (5th index)1/1 -> InternalMechanics/2(Velocity), Bus Creator1/2  "velocity"
  PS-Simulink Converter2/1 -> Gain2/1
  Constant2/1 -> Assignment (5th index)2/1
  Gain2/1 -> Assignment (5th index)2/2
  Constant3/1 -> Assignment (5th index)3/1
  Gain3/1 -> Assignment (5th index)3/2
  PS-Simulink Converter3/1 -> Gain3/1
  Assignment (5th index)2/1 -> Bus Creator1/3  "acceleration"
  Assignment (5th index)3/1 -> Bus Creator1/5  "forceActuation"
  InternalMechanics/1(Force) -> Bus Creator1/7  "forceInternalMechanics"
  InternalMechanics/2(Power) -> Bus Creator1/8  "powerInternal Mechanics"
  connections:
  F/RConn1 -- Rigid Transform1/LConn1
  B/RConn1 -- Rigid Transform/LConn1
  Pitch PCC (Revolute Joint)/LConn1 -- Rigid Transform/RConn1
  Pitch PCC (Revolute Joint)/RConn1 -- Rigid Transform1/RConn1
  PS-Simulink Converter7/LConn1 -- Pitch PCC (Revolute Joint)/RConn9
  PS-Simulink Converter6/LConn1 -- Pitch PCC (Revolute Joint)/RConn8
  PS-Simulink Converter5/LConn1 -- Pitch PCC (Revolute Joint)/RConn7
  PS-Simulink Converter4/LConn1 -- Pitch PCC (Revolute Joint)/RConn6
  Pitch PCC (Revolute Joint)/RConn2 -- PS-Simulink Converter/LConn1
  Pitch PCC (Revolute Joint)/RConn3 -- PS-Simulink Converter1/LConn1
  PS-Simulink Converter2/LConn1 -- Pitch PCC (Revolute Joint)/RConn4
  PS-Simulink Converter3/LConn1 -- Pitch PCC (Revolute Joint)/RConn5

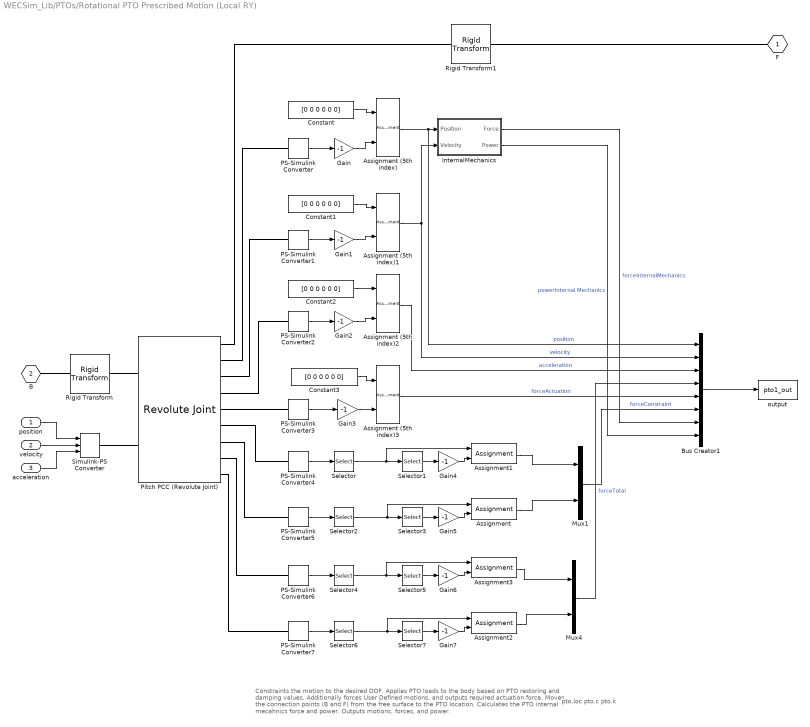
== system WECSim_Lib/PTOs/Rotational PTO Prescribed Motion (Local RY) ==
  note: Constraints the motion to the desired DOF.
      | Applies PTO loads to the body based on PTO restoring and damping values.
      | Additionally forces User Defined motions, and outputs required actuation force.
      | Moves the connection points (B and F) from the free surface to the PTO location.
      | Calculates the PTO internal mecahnics force and power.
      | Outputs motions, forces, and power.
  note: pto.loc
      | pto.c
      | pto.k
  position : Inport
  velocity : Inport  Port=2
  acceleration : Inport  Port=3
  Assignment{,1..3} (4 alike) : Assignment  DiagnosticForDimensions=Warning  Indices=2
  "Assignment (5th index) " : Assignment  Indices=5
  Assignment (5th index)1 : Assignment  Indices=5
  Assignment (5th index)2 : Assignment  Indices=5
  Assignment (5th index)3 : Assignment  Indices=5
  Bus Creator1 : BusCreator  Inputs=8
  Constant{,1..3} (4 alike) : Constant  Value=[0 0 0 0 0 0]
  Gain{,1..7} (8 alike) : Gain  Gain=-1
  InternalMechanics : Subsystem
  Mux1 : Mux  Inputs=2
  Mux4 : Mux  Inputs=2
  PS-Simulink Converter{,1..7} (8 alike) : nesl_utility/PS-Simulink Converter  PhysicalDomain=network_engine_domain  SubClassName=ps_output  LeftPortType=input  RightPortType=output  PseudoPeriodic=off  Frequencies=[]  Unit=1  AffineConversion=off
  Pitch PCC (Revolute Joint) : sm_lib/Joints/Revolute Joint  SenseConstraintForce=on  SenseConstraintForceX=off  SenseConstraintForceY=off  SenseConstraintForceZ=off  SenseConstraintTorque=on  SenseConstraintTorqueX=off  SenseConstraintTorqueY=off  SenseConstraintTorqueZ=off  SenseTotalForce=on  SenseTotalForceX=off  SenseTotalForceY=off  SenseTotalForceZ=off  SenseTotalTorque=on  SenseTotalTorqueX=off  SenseTotalTorqueY=off  SenseTotalTorqueZ=off  CompositeWrenchDir=BaseOnFollower  CompositeWrenchFrame=BaseFrame  EquilibriumPosition=0  EquilibriumPositionUnits=deg  SpringStiffness=pto.k  SpringStiffnessUnits=N*m/rad  DampingCoefficient=pto.c  DampingCoefficientUnits=N*m/(rad/s)  TorqueActuationMode=ComputedTorque  MotionActuationMode=InputMotion  SensePosition=on  SenseVelocity=on  SenseAcceleration=on  SenseTorqueForce=on  PositionTargetValue=0  PositionTargetValueUnits=deg  PositionTargetSpecify=off  PositionTargetPriority=High  VelocityTargetValue=0  VelocityTargetValueUnits=deg/s  VelocityTargetSpecify=off  VelocityTargetPriority=High  BlockFunction=simmechanics.library.joints.revolute_joint
  Rigid Transform : sm_lib/Frames and Transforms/Rigid Transform  TranslationMethod=Cartesian  TranslationLengthUnit=m  TranslationStandardAxis=+Z  TranslationStandardOffset=0  TranslationCartesianOffset=pto.loc  TranslationROffset=0  TranslationROffsetUnits=m  TranslationZOffset=0  TranslationZOffsetUnits=m  TranslationThetaOffset=0  TranslationThetaOffsetUnits=deg  RotationMethod=StandardAxis  RotationAngleUnits=deg  RotationStandardAxis=+X  RotationAngle=90  RotationArbitraryAxis=[0 0 1]  FollAlignAxisA=+X  BaseAlignAxisA=+Y  FollAlignAxisB=+Y  BaseAlignAxisB=+Z  RotationMatrix=[1 0 0; 0 1 0; 0 0 1]  BlockFunction=simmechanics.library.frames_transforms.rigid_transform
  Rigid Transform1 : sm_lib/Frames and Transforms/Rigid Transform  TranslationMethod=Cartesian  TranslationLengthUnit=m  TranslationStandardAxis=+Z  TranslationStandardOffset=0  TranslationCartesianOffset=pto.loc  TranslationROffset=0  TranslationROffsetUnits=m  TranslationZOffset=0  TranslationZOffsetUnits=m  TranslationThetaOffset=0  TranslationThetaOffsetUnits=deg  RotationMethod=StandardAxis  RotationAngleUnits=deg  RotationStandardAxis=+X  RotationAngle=90  RotationArbitraryAxis=[0 0 1]  FollAlignAxisA=+X  BaseAlignAxisA=+Y  FollAlignAxisB=+Y  BaseAlignAxisB=+Z  RotationMatrix=[1 0 0; 0 1 0; 0 0 1]  BlockFunction=simmechanics.library.frames_transforms.rigid_transform
  Selector{,2,4,6} (4 alike) : Selector  InputPortWidth=3  Indices=[1 3 2]
  Selector{1,3,5,7} (4 alike) : Selector  InputPortWidth=3  Indices=[2]
  Simulink-PS Converter : nesl_utility/Simulink-PS Converter  PhysicalDomain=network_engine_domain  SubClassName=ps_input  LeftPortType=input  RightPortType=output  PseudoPeriodic=off  Frequencies=[]  NoiseDistribution=none  NoiseParameters=[]  Unit=1  AffineConversion=off  InputFiltering=derivs  SimscapeFilterOrder=2  InputFilterTimeConstant=0.001  UdotUserProvided=2
  output : ToWorkspace  VariableName=pto1_out  SaveFormat=Structure With Time  SampleTime=-1
      settings: Decimation=round(simu.dtOut/simu.dt,0)
  F : PMIOPort  Port=1  Side=Left
  B : PMIOPort  Port=2  Side=Right
  wires:
  InternalMechanics/2(Power) -> Bus Creator1/8  "powerInternal Mechanics"
  InternalMechanics/1(Force) -> Bus Creator1/7  "forceInternalMechanics"
  Assignment (5th index)3/1 -> Bus Creator1/5  "forceActuation"
  Assignment (5th index)2/1 -> Bus Creator1/3  "acceleration"
  PS-Simulink Converter3/1 -> Gain3/1
  Gain3/1 -> Assignment (5th index)3/2
  Constant3/1 -> Assignment (5th index)3/1
  Gain2/1 -> Assignment (5th index)2/2
  Constant2/1 -> Assignment (5th index)2/1
  PS-Simulink Converter2/1 -> Gain2/1
  Assignment (5th index)1/1 -> InternalMechanics/2(Velocity), Bus Creator1/2  "velocity"
  PS-Simulink Converter1/1 -> Gain1/1
  Gain1/1 -> Assignment (5th index)1/2
  Constant1/1 -> Assignment (5th index)1/1
  "Assignment (5th index) "/1 -> InternalMechanics/1(Position), Bus Creator1/1  "position"
  Gain/1 -> "Assignment (5th index) "/2
  PS-Simulink Converter/1 -> Gain/1
  Constant/1 -> "Assignment (5th index) "/1
  Assignment3/1 -> Mux4/1
  Assignment2/1 -> Mux4/2
  PS-Simulink Converter7/1 -> Selector6/1
  PS-Simulink Converter6/1 -> Selector4/1
  Gain6/1 -> Assignment3/2
  Selector5/1 -> Gain6/1
  Selector4/1 -> Assignment3/1, Selector5/1
  Gain7/1 -> Assignment2/2
  Selector7/1 -> Gain7/1
  Selector6/1 -> Assignment2/1, Selector7/1
  Mux4/1 -> Bus Creator1/4  "forceTotal"
  Bus Creator1/1 -> output/1
  PS-Simulink Converter4/1 -> Selector/1
  PS-Simulink Converter5/1 -> Selector2/1
  Mux1/1 -> Bus Creator1/6  "forceConstraint"
  Assignment1/1 -> Mux1/1
  Assignment/1 -> Mux1/2
  Gain4/1 -> Assignment1/2
  Selector1/1 -> Gain4/1
  Selector/1 -> Selector1/1, Assignment1/1
  Gain5/1 -> Assignment/2
  Selector3/1 -> Gain5/1
  Selector2/1 -> Selector3/1, Assignment/1
  acceleration/1 -> Simulink-PS Converter/3
  velocity/1 -> Simulink-PS Converter/2
  position/1 -> Simulink-PS Converter/1
  connections:
  PS-Simulink Converter5/LConn1 -- Pitch PCC (Revolute Joint)/RConn7
  PS-Simulink Converter4/LConn1 -- Pitch PCC (Revolute Joint)/RConn6
  PS-Simulink Converter2/LConn1 -- Pitch PCC (Revolute Joint)/RConn4
  Pitch PCC (Revolute Joint)/RConn1 -- Rigid Transform1/RConn1
  B/RConn1 -- Rigid Transform/LConn1
  Pitch PCC (Revolute Joint)/LConn1 -- Rigid Transform/RConn1
  Pitch PCC (Revolute Joint)/RConn2 -- PS-Simulink Converter/LConn1
  Pitch PCC (Revolute Joint)/RConn3 -- PS-Simulink Converter1/LConn1
  F/RConn1 -- Rigid Transform1/LConn1
  PS-Simulink Converter7/LConn1 -- Pitch PCC (Revolute Joint)/RConn9
  PS-Simulink Converter6/LConn1 -- Pitch PCC (Revolute Joint)/RConn8
  PS-Simulink Converter3/LConn1 -- Pitch PCC (Revolute Joint)/RConn5
  Pitch PCC (Revolute Joint)/LConn2 -- Simulink-PS Converter/RConn1

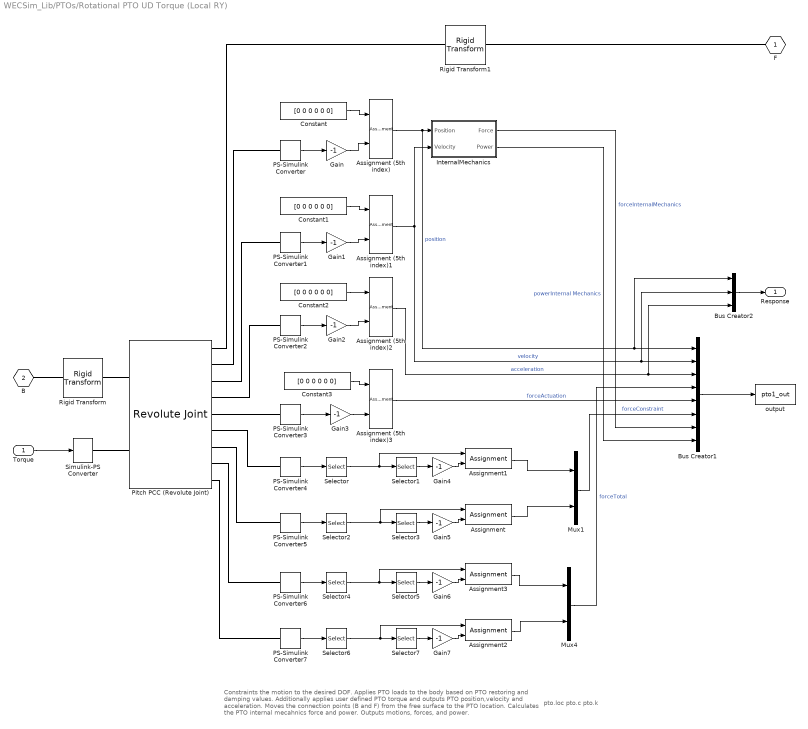
== system WECSim_Lib/PTOs/Rotational PTO UD Torque (Local RY) ==
  note: pto.loc
      | pto.c
      | pto.k
  note: Constraints the motion to the desired DOF.
      | Applies PTO loads to the body based on PTO restoring and damping values.
      | Additionally applies user defined PTO torque and outputs PTO position,velocity and acceleration.
      | Moves the connection points (B and F) from the free surface to the PTO location.
      | Calculates the PTO internal mecahnics force and power.
      | Outputs motions, forces, and power.
  Torque : Inport
  Assignment{,1..3} (4 alike) : Assignment  DiagnosticForDimensions=Warning  Indices=2
  "Assignment (5th index) " : Assignment  Indices=5
  Assignment (5th index)1 : Assignment  Indices=5
  Assignment (5th index)2 : Assignment  Indices=5
  Assignment (5th index)3 : Assignment  Indices=5
  Bus Creator1 : BusCreator  Inputs=8
  Bus Creator2 : BusCreator  Inputs=3
  Constant{,1..3} (4 alike) : Constant  Value=[0 0 0 0 0 0]
  Gain{,1..7} (8 alike) : Gain  Gain=-1
  InternalMechanics : Subsystem
  Mux1 : Mux  Inputs=2
  Mux4 : Mux  Inputs=2
  PS-Simulink Converter{,1..7} (8 alike) : nesl_utility/PS-Simulink Converter  PhysicalDomain=network_engine_domain  SubClassName=ps_output  LeftPortType=input  RightPortType=output  PseudoPeriodic=off  Frequencies=[]  Unit=1  AffineConversion=off
  Pitch PCC (Revolute Joint) : sm_lib/Joints/Revolute Joint  SenseConstraintForce=on  SenseConstraintForceX=off  SenseConstraintForceY=off  SenseConstraintForceZ=off  SenseConstraintTorque=on  SenseConstraintTorqueX=off  SenseConstraintTorqueY=off  SenseConstraintTorqueZ=off  SenseTotalForce=on  SenseTotalForceX=off  SenseTotalForceY=off  SenseTotalForceZ=off  SenseTotalTorque=on  SenseTotalTorqueX=off  SenseTotalTorqueY=off  SenseTotalTorqueZ=off  CompositeWrenchDir=BaseOnFollower  CompositeWrenchFrame=BaseFrame  EquilibriumPosition=0  EquilibriumPositionUnits=deg  SpringStiffness=pto.k  SpringStiffnessUnits=N*m/rad  DampingCoefficient=pto.c  DampingCoefficientUnits=N*m/(rad/s)  TorqueActuationMode=InputTorque  MotionActuationMode=ComputedMotion  SensePosition=on  SenseVelocity=on  SenseAcceleration=on  SenseTorqueForce=on  PositionTargetValue=0  PositionTargetValueUnits=deg  PositionTargetSpecify=off  PositionTargetPriority=High  VelocityTargetValue=0  VelocityTargetValueUnits=deg/s  VelocityTargetSpecify=off  VelocityTargetPriority=High  BlockFunction=simmechanics.library.joints.revolute_joint
  Rigid Transform : sm_lib/Frames and Transforms/Rigid Transform  TranslationMethod=Cartesian  TranslationLengthUnit=m  TranslationStandardAxis=+Z  TranslationStandardOffset=0  TranslationCartesianOffset=pto.loc  TranslationROffset=0  TranslationROffsetUnits=m  TranslationZOffset=0  TranslationZOffsetUnits=m  TranslationThetaOffset=0  TranslationThetaOffsetUnits=deg  RotationMethod=StandardAxis  RotationAngleUnits=deg  RotationStandardAxis=+X  RotationAngle=90  RotationArbitraryAxis=[0 0 1]  FollAlignAxisA=+X  BaseAlignAxisA=+Y  FollAlignAxisB=+Y  BaseAlignAxisB=+Z  RotationMatrix=[1 0 0; 0 1 0; 0 0 1]  BlockFunction=simmechanics.library.frames_transforms.rigid_transform
  Rigid Transform1 : sm_lib/Frames and Transforms/Rigid Transform  TranslationMethod=Cartesian  TranslationLengthUnit=m  TranslationStandardAxis=+Z  TranslationStandardOffset=0  TranslationCartesianOffset=pto.loc  TranslationROffset=0  TranslationROffsetUnits=m  TranslationZOffset=0  TranslationZOffsetUnits=m  TranslationThetaOffset=0  TranslationThetaOffsetUnits=deg  RotationMethod=StandardAxis  RotationAngleUnits=deg  RotationStandardAxis=+X  RotationAngle=90  RotationArbitraryAxis=[0 0 1]  FollAlignAxisA=+X  BaseAlignAxisA=+Y  FollAlignAxisB=+Y  BaseAlignAxisB=+Z  RotationMatrix=[1 0 0; 0 1 0; 0 0 1]  BlockFunction=simmechanics.library.frames_transforms.rigid_transform
  Selector{,2,4,6} (4 alike) : Selector  InputPortWidth=3  Indices=[1 3 2]
  Selector{1,3,5,7} (4 alike) : Selector  InputPortWidth=3  Indices=[2]
  Simulink-PS Converter : nesl_utility/Simulink-PS Converter  PhysicalDomain=network_engine_domain  SubClassName=ps_input  LeftPortType=input  RightPortType=output  PseudoPeriodic=off  Frequencies=[]  NoiseDistribution=none  NoiseParameters=[]  Unit=1  AffineConversion=off  InputFiltering=off  SimscapeFilterOrder=1  InputFilterTimeConstant=0.001  UdotUserProvided=1
  output : ToWorkspace  VariableName=pto1_out  SaveFormat=Structure With Time  SampleTime=-1
      settings: Decimation=round(simu.dtOut/simu.dt,0)
  F : PMIOPort  Port=1  Side=Left
  B : PMIOPort  Port=2  Side=Right
  Response : Outport
  wires:
  InternalMechanics/2(Power) -> Bus Creator1/8  "powerInternal Mechanics"
  InternalMechanics/1(Force) -> Bus Creator1/7  "forceInternalMechanics"
  Assignment (5th index)3/1 -> Bus Creator1/5  "forceActuation"
  Assignment (5th index)2/1 -> Bus Creator1/3, Bus Creator2/3  "acceleration"
  PS-Simulink Converter3/1 -> Gain3/1
  Gain3/1 -> Assignment (5th index)3/2
  Constant3/1 -> Assignment (5th index)3/1
  Gain2/1 -> Assignment (5th index)2/2
  Constant2/1 -> Assignment (5th index)2/1
  PS-Simulink Converter2/1 -> Gain2/1
  Assignment (5th index)1/1 -> InternalMechanics/2(Velocity), Bus Creator1/2, Bus Creator2/2  "velocity"
  PS-Simulink Converter1/1 -> Gain1/1
  Gain1/1 -> Assignment (5th index)1/2
  Constant1/1 -> Assignment (5th index)1/1
  "Assignment (5th index) "/1 -> InternalMechanics/1(Position), Bus Creator1/1, Bus Creator2/1  "position"
  Gain/1 -> "Assignment (5th index) "/2
  PS-Simulink Converter/1 -> Gain/1
  Constant/1 -> "Assignment (5th index) "/1
  Assignment3/1 -> Mux4/1
  Assignment2/1 -> Mux4/2
  PS-Simulink Converter7/1 -> Selector6/1
  PS-Simulink Converter6/1 -> Selector4/1
  Gain6/1 -> Assignment3/2
  Selector5/1 -> Gain6/1
  Selector4/1 -> Assignment3/1, Selector5/1
  Gain7/1 -> Assignment2/2
  Selector7/1 -> Gain7/1
  Selector6/1 -> Assignment2/1, Selector7/1
  Mux4/1 -> Bus Creator1/4  "forceTotal"
  Bus Creator1/1 -> output/1
  PS-Simulink Converter4/1 -> Selector/1
  PS-Simulink Converter5/1 -> Selector2/1
  Mux1/1 -> Bus Creator1/6  "forceConstraint"
  Assignment1/1 -> Mux1/1
  Assignment/1 -> Mux1/2
  Gain4/1 -> Assignment1/2
  Selector1/1 -> Gain4/1
  Selector/1 -> Selector1/1, Assignment1/1
  Gain5/1 -> Assignment/2
  Selector3/1 -> Gain5/1
  Selector2/1 -> Selector3/1, Assignment/1
  Torque/1 -> Simulink-PS Converter/1
  Bus Creator2/1 -> Response/1
  connections:
  PS-Simulink Converter5/LConn1 -- Pitch PCC (Revolute Joint)/RConn7
  PS-Simulink Converter4/LConn1 -- Pitch PCC (Revolute Joint)/RConn6
  PS-Simulink Converter2/LConn1 -- Pitch PCC (Revolute Joint)/RConn4
  Pitch PCC (Revolute Joint)/RConn1 -- Rigid Transform1/RConn1
  B/RConn1 -- Rigid Transform/LConn1
  Pitch PCC (Revolute Joint)/LConn1 -- Rigid Transform/RConn1
  Pitch PCC (Revolute Joint)/RConn2 -- PS-Simulink Converter/LConn1
  Pitch PCC (Revolute Joint)/RConn3 -- PS-Simulink Converter1/LConn1
  F/RConn1 -- Rigid Transform1/LConn1
  PS-Simulink Converter7/LConn1 -- Pitch PCC (Revolute Joint)/RConn9
  PS-Simulink Converter6/LConn1 -- Pitch PCC (Revolute Joint)/RConn8
  PS-Simulink Converter3/LConn1 -- Pitch PCC (Revolute Joint)/RConn5
  Simulink-PS Converter/RConn1 -- Pitch PCC (Revolute Joint)/LConn2
